simulink model "model_SEIRD"  (R2023a)
settings: Solver=VariableStepAuto  StartTime=0.0  StopTime=365.00  RelTol=1e-3
model workspace (MAT data in the model file):
  b = 0.3
  d = 0.02
  g = 0.1
  l = 0.2
  n = 7700000
settings Model: Creator=joans  LastModifiedBy=joans
settings ModelReferenceCC: EnableRefExpFcnMdlSchedulingChecks=on

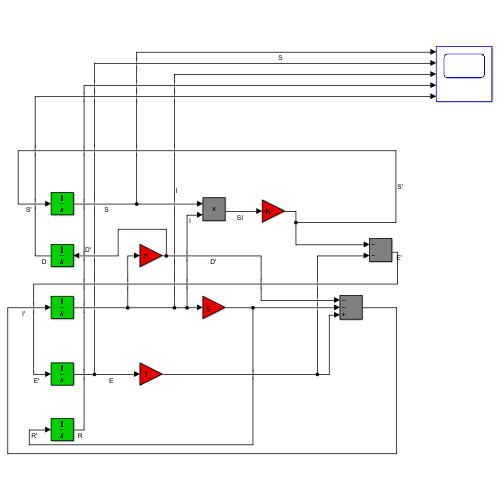
[thumbnail: Simulink's stored preview of the top-level diagram]
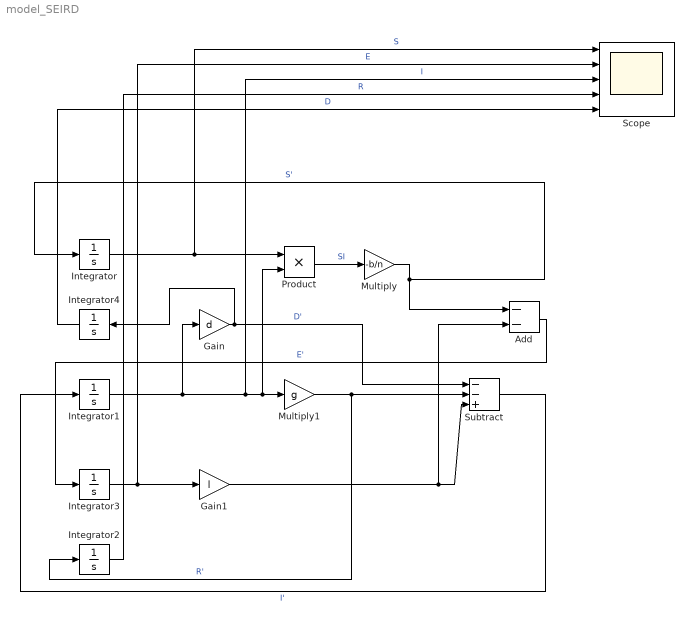
== system model_SEIRD ==
  Add : Sum  Inputs=--
  Gain : Gain  Gain=d
  Gain1 : Gain  Gain=l
  Integrator : Integrator  InitialCondition=n
  Integrator1 : Integrator  InitialCondition=1000
  Integrator2 : Integrator
  Integrator3 : Integrator
  Integrator4 : Integrator
  Multiply : Gain  Gain=-b/n
  Multiply1 : Gain  Gain=g
  Product : Product
  Scope : Scope  NumInputPorts=5
  Subtract : Sum  Inputs=--+
  wires:
  Integrator/1 -> Scope/1, Product/1  "S"
  Integrator1/1 -> Scope/3, Product/2, Multiply1/1, Gain/1  "I"
  Product/1 -> Multiply/1  "SI"
  Multiply/1 -> Add/1, Integrator/1  "S'"
  Multiply1/1 -> Integrator2/1, Subtract/2  "R'"
  Integrator2/1 -> Scope/4  "R"
  Integrator3/1 -> Scope/2, Gain1/1  "E"
  Subtract/1 -> Integrator1/1  "I'"
  Integrator4/1 -> Scope/5  "D"
  Gain/1 -> Integrator4/1, Subtract/1  "D'"
  Gain1/1 -> Add/2, Subtract/3
  Add/1 -> Integrator3/1  "E'"
